simulink library "cdsIPCS"  (Simulink 7.0)
settings Model: Creator=Rolf  LastModifiedBy=Rolf

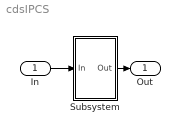
== system cdsIPCS ==
  In : Inport  OutDataType=sfix(16)  OutScaling=2^0
  Subsystem : Subsystem
  Out : Outport  OutDataType=sfix(16)  OutScaling=2^0
  wires:
  Subsystem/1(Out) -> Out/1
  In/1 -> Subsystem/1(In)

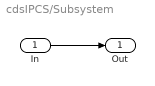
== system cdsIPCS/Subsystem ==
  In : Inport  OutDataType=sfix(16)  OutScaling=2^0
  Out : Outport  OutDataType=sfix(16)  OutScaling=2^0
  wires:
  In/1 -> Out/1
